simulink model "BMSSOCEstimation"  (R2025b)
settings: Solver=FixedStepDiscrete  StartTime=0.0  StopTime=10000  FixedStep=0.1  RelTol=1e-3
model workspace (MAT data in the model file):
  Battery.SOC_LUT = [0.01 0.02 0.03 0.04 0.05 0.06 0.07 0.08 0.09 0.1 0.11 0.12 0.13 0.14 0.15 0.16 0.17 0.18 0.19 0.2 0.21 0.22 0.23 0.24 0.25 0.26 0.27 0.28 0.29 0.3 0.31 0.32 0.33 0.34 0.35 0.36 0.37 0.38 0.39 0.4 0.41 0.42 0.43 0.44 0.45 0.46 0.47 0.48 0.49 0.5 0.51 0.52 0.53 0.54 0.55 0.56 0.57 0.58 0.59 0.6 0.61 0.62 0.63 0.64 0.65 0.66 0.67 0.68 0.69 0.7 0.71 0.72 0.73 0.74 0.75 0.76 0.77 0.78 0.79 0.8 0.81 0.82 0.83 0.84 0.85 0.86 0.87 0.88 0.89 0.9 0.91 0.92 0.93 0.94 0.95 0.96 0.97 0.98 0.99 1]
  Battery.Temperature_LUT = [-10 0 25 40]
  Battery.Capacity_LUT = [4.04528301887 4.19622641509 4.8 4.73962264151]
  Battery.Em_LUT = [2.67308083891 2.74411674384 2.80408613071 2.86247711994 2.90851059763 2.94904306488 2.9829846776 3.01467102589 3.04031502638 3.06256828113 3.08180972392 3.09994219643 ... (400 elements, 100x4)]
  Battery.R0_LUT = [0.0569026752707 0.0575506938969 0.0576730924021 0.0575627404981 0.0573787336615 0.0571931123197 0.0568199985482 0.056411926464 0.0561974340667 0.0560805640861 0.0557640899305 0.055275807865 ... (400 elements, 100x4)]
  Battery.R1_LUT = [0.0035 0.0035 0.0035 0.0035 0.0035 0.0035 0.0035 0.0035 0.0035 0.0035 0.0035 0.0035 ... (400 elements, 100x4)]
  Battery.C1_LUT = [5000 5000 5000 5000 5000 5000 5000 5000 5000 5000 5000 5000 ... (400 elements, 100x4)]
  Battery.Mass = 0.047
  Battery.ThermalMass = 44
  Battery.R_bleed = 20
  Battery.h_conv = 5
  Battery.cell_area = 0.0037
  Battery.TempInit = 25
  Battery.SOCInit = 0.75
  Battery.Model = 'panasonic ncr18650bd'
  Battery.DischargeCycle_LUT = [1 5 9 13 17 21 25 29 33 37 41 45 49 53 57 61 65 69 73 77 81 85 89 93 97 101 105 109 113 117 121 125 129 133 137 141 145 149 153 157 161 165 169 173 177 181 185 189 193 197 201 205 209 213 217 221 225 229 233 237 241 245 249 253 257 261 265 269 273 277 281 285 289 293 297 301 305 309 313 317]
  Battery.deltaEm_LUT = [0 -0.363115641304 -0.600096647258 -0.689070000839 -0.76773380251 -0.846397604181 -0.926368385458 -0.992711297521 -1.05704974111 -1.12227693902 -1.19018070587 -1.25808447272 -1.31699459748 -1.35876443799 -1.40168267642 -1.44460091485 -1.48751915327 -1.5304373917 -1.57335563013 -1.62198241593 -1.67232184498 -1.71858340023 -1.76179802551 -1.8050126508 -1.84822727608 -1.8917937136 -1.93575272784 -1.97971174208 -2.02367075632 -2.06762977056 -2.11171979109 -2.15588700406 -2.19980020032 -2.24365853098 -2.28751686164 -2.33137519231 -2.37523352297 -2.41909185363 -2.45982559031 -2.49599372373 -2.53216185715 -2.56832999058 -2.604498124 -2.64066625743 -2.67683439085 -2.71300252428 -2.7491706577 -2.78367585394 -2.81632179346 -2.8483348579 -2.88034792233 -2.91236098677 -2.94437405121 -2.97638711564 -3.00840018008 -3.04041324451 -3.07260346059 -3.10359008254 -3.13082308991 -3.15805609728 -3.18528910464 -3.21252211201 -3.23975511938 -3.26698812675 -3.29422113412 -3.32122400938 -3.3463475604 -3.37152613073 -3.39670470105 -3.42188327138 -3.4470618417 -3.47224041203 -3.49938358795 -3.52900276724 -3.55862194653 -3.58824112582 -3.6178603051 -3.64748858268 -3.67711690909 -3.70674523549]
  Battery.deltaCapacity_LUT = [0 -0.860019120059 -1.71332421702 -2.0819400264 -2.45055583577 -2.81917164515 -3.18778745452 -3.48884924257 -3.7808148236 -4.07278040463 -4.36474598566 -4.6567115667 -4.91000721732 -5.08494410056 -5.2598809838 -5.43481786703 -5.60975475027 -5.78469163351 -5.95962851674 -6.13456539998 -6.30950228322 -6.47026795816 -6.62044510558 -6.77062225299 -6.92079940041 -7.07097654783 -7.22115369524 -7.37133084266 -7.52150799007 -7.67168513749 -7.82230984162 -7.97319825819 -8.12408667477 -8.27497509134 -8.42586350792 -8.57675192449 -8.72764034107 -8.87852875764 -9.01789522921 -9.13717923376 -9.25646323831 -9.37574724285 -9.4950312474 -9.61431525195 -9.73359925649 -9.85288326104 -9.97216726558 -10.0914512701 -10.2059878191 -10.3183039593 -10.4306200996 -10.5429362398 -10.65525238 -10.7675685203 -10.8798846605 -10.9922008008 -11.104516941 -11.2125891929 -11.3075699376 -11.4025506823 -11.4975314271 -11.5925121718 -11.6874929166 -11.7824736613 -11.877454406 -11.9716325175 -12.0588579537 -12.1460833899 -12.2333088261 -12.3205342623 -12.4077596986 -12.4949851348 -12.5890165008 -12.6916254178 -12.7942343349 -12.8968432519 -12.999452169 -13.102061086 -13.2046700031 -13.3072789201]
  Battery.cond_thickness = 0.001
  Battery.thermal_conductivity = 205
  Ts = Simulink.Parameter
  Ts.Value = 0.1
  Ts.Complexity = 'real'
  Ts.Dimensions = [1 1]
  Ts.DataType = 'double'
undefined symbols (not defined in the file): DiscIntNeverNeededParam, PlntBattNumCellPar, PlntBattSocInit
libraries: sharedTrackingLibrary x2, simulink x1
settings Model: DataDictionary=VirtualMotoTemplate.sldd  ModifiedByFormat=The MathWorks, Inc.  ExtModeTrigDuration=5  Creator=The MathWorks, Inc.  LastModifiedBy=The MathWorks, Inc.
settings SolverCC: AlgebraicLoopSolver=TrustRegion  PositivePriorityOrder=on  AutoInsertRateTranBlk=on  MaxZcPerStep=1.0
settings DataIOCC: ExternalInput=Battery  SaveOutput=off  SaveTime=off  SignalLoggingName=logsOut
settings OptimizationCC: BlockReduction=off  DefaultParameterBehavior=Inlined  UseFloatMulNetSlope=on  DefaultUnderspecifiedDataType=single  OptimizeBlockIOStorage=off  ReuseModelBlockBuffer=off  EnhancedBackFolding=on  PassReuseOutputArgsThreshold=0.0  ZeroExternalMemoryAtStartup=off  ZeroInternalMemoryAtStartup=off  EfficientFloat2IntCast=on  MaxStackSize=64  OptimizeBlockOrder=speed  DifferentSizesBufferReuse=on
settings DebuggingCC: SignalInfNanChecking=error  SaveWithParameterizedLinksMsg=none  CheckExecutionContextPreStartOutputMsg=on  IntegerOverflowMsg=error  ParameterPrecisionLossMsg=none  ParameterTunabilityLossMsg=error  UnconnectedInputMsg=warning  UnconnectedOutputMsg=warning  UnconnectedLineMsg=warning  AssertControl=DisableAll  PregeneratedLibrarySubsystemCodeDiagnostic=none  SFUnexpectedBacktrackingDiag=warning  SFNoUnconditionalDefaultTransitionDiag=warning  SFExecutionAtInitializationDiag=none  ArithmeticOperatorsInVariantConditions=warning
settings HardwareCC: ProdBitPerLong=64.0  ProdLongLongMode=on  ProdHWDeviceType=Intel->x86-64 (Linux 64)
settings ModelReferenceCC: EnableRefExpFcnMdlSchedulingChecks=on  ModelReferenceNumInstancesAllowed=Single  PropagateSignalLabelsOutOfModel=off
settings SFSimCC: SimUseLocalCustomCode=off  MATLABDynamicMemAlloc=off  CustomCodeUndefinedFunction=UseInterfaceOnly
settings RTWCC: GenerateReport=on  RTWUseLocalCustomCode=off  Toolchain=Simulink Real-Time Toolchain  BuildConfiguration=Faster Runs  TargetLang=C++  GPUComputeCapability=3.5  DLArmComputeVersion=19.05
settings CodeAppCC: ForceParamTrailComments=on  MaxIdLength=51.0  OperatorAnnotations=on  MangleLength=4.0
settings GRTTargetCC: TargetLangStandard=C++03 (ISO)  CodeInterfacePackaging=C++ class  SubcomponentCodeInterfacePackaging=C++ class
settings ConfigComp: CovMetricSettings=dcw  CovSaveCumulativeToWorkspaceVar=on  CovSaveSingleToWorkspaceVar=on  CovExternalEMLEnable=off  CovSFcnEnable=off  DVMode=DesignErrorDetection  DVMaxProcessTime=7000.0  DVMaxTestCaseSteps=10000.0  DVTestSuiteOptimization=Auto  DVAbsoluteTolerance=1.0e-5  DVDefectChecker=on  DVDetectDeadLogic=on  DVDetectIntegerOverflow=off  DVMaxViolationSteps=20.0  DVHarnessSource=Signal Editor  DVRebuildModelRepresentation=Always  DVActiveTab=0.0

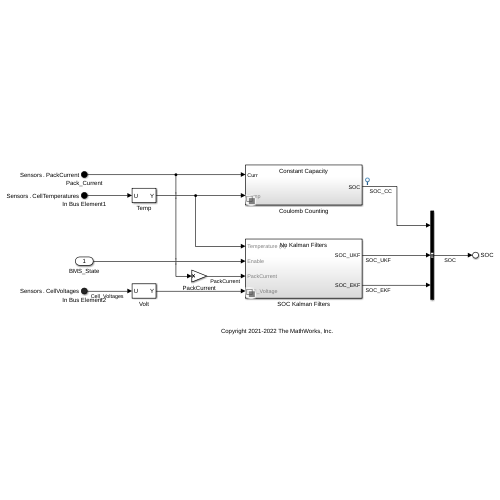
[thumbnail: Simulink's stored preview of the top-level diagram]
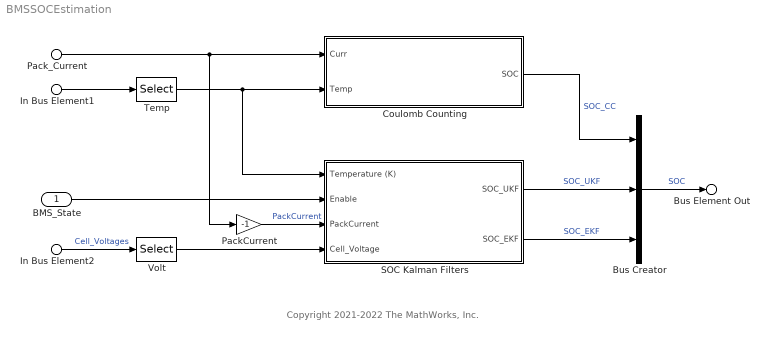
== system BMSSOCEstimation ==
  note: Copyright 2021-2022 The MathWorks, Inc.
  BMS_State : Inport
  In Bus Element2 : Inport  Port=2  PortName=Sensors  Element=CellVoltages
  Pack_Current : Inport  Port=2  PortName=Sensors  Element=PackCurrent
  In Bus Element1 : Inport  Port=2  PortName=Sensors  Element=CellTemperatures
  Bus Creator : BusCreator  Inputs=3
  Coulomb Counting : Subsystem  Variant=on  VariantControlMode=label  VariantControl=SocAlgo==1  LabelModeActiveChoice=Constant Capacity
  PackCurrent : Gain  Gain=-1
  SOC Kalman Filters : Subsystem  Variant=on  VariantControlMode=label  VariantControl=Choice  LabelModeActiveChoice=No Kalman Filters
  Temp : Selector  InputPortWidth=PlntBattNumCellSer  IndexOptions=Index vector (dialog)  Indices=1  OutputSizes=1
  Volt : Selector  InputPortWidth=PlntBattNumCellSer  IndexOptions=Index vector (dialog)  Indices=1  OutputSizes=1
  Bus Element Out : Outport  PortName=SOC
  wires:
  Bus Creator/1 -> Bus Element Out/1  "SOC"
  In Bus Element2/1 -> Volt/1  "Cell_Voltages"
  Temp/1 -> Coulomb Counting/2(Temp), SOC Kalman Filters/1(Temperature (K))
  Pack_Current/1 -> Coulomb Counting/1(Curr), PackCurrent/1
  In Bus Element1/1 -> Temp/1
  Coulomb Counting/1(SOC) -> Bus Creator/1  "SOC_CC"
  BMS_State/1 -> SOC Kalman Filters/2(Enable)
  PackCurrent/1 -> SOC Kalman Filters/3(PackCurrent)  "PackCurrent"
  Volt/1 -> SOC Kalman Filters/4(Cell_Voltage)
  SOC Kalman Filters/1(SOC_UKF) -> Bus Creator/2  "SOC_UKF"
  SOC Kalman Filters/2(SOC_EKF) -> Bus Creator/3  "SOC_EKF"

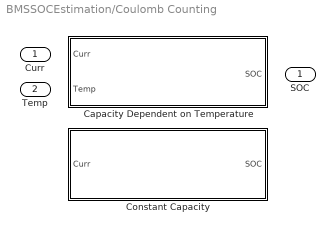
== system BMSSOCEstimation/Coulomb Counting ==
  Curr : Inport
  Temp : Inport  Port=2
  Capacity Dependent on Temperature : Subsystem  VariantControl=Capacity Dependent on Temperature
  Constant Capacity : Subsystem  VariantControl=Constant Capacity
  SOC : Outport

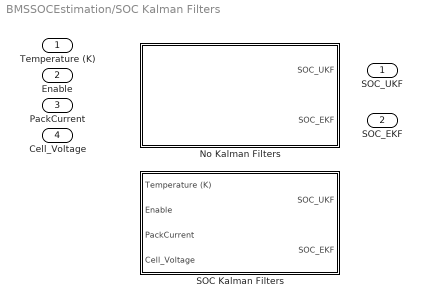
== system BMSSOCEstimation/SOC Kalman Filters ==
  Temperature (K) : Inport
  Enable : Inport  Port=2
  PackCurrent : Inport  Port=3
  Cell_Voltage : Inport  Port=4
  No Kalman Filters : Subsystem  VariantControl=No Kalman Filters
  SOC Kalman Filters : Subsystem  InitFcn=|  VariantControl=SOC Kalman Filters
      | if ~license('test', 'identification_toolbox') 
      |   error(['Block' gcb ' Requires System Identification Toolbox']) 
      | end 
      | 
      | if ~license('test', 'control_toolbox') 
      |     error(['Block' gcb ' Requires Control System Toolbox']) 
      | end
  SOC_UKF : Outport
  SOC_EKF : Outport  Port=2

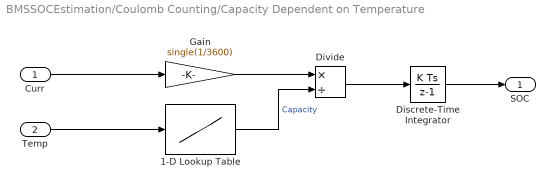
== system BMSSOCEstimation/Coulomb Counting/Capacity Dependent on Temperature ==
  Curr : Inport
  Temp : Inport  Port=2
  1-D Lookup Table : Lookup_n-D  NumberOfTableDimensions=1  BreakpointsForDimension1=single(Battery(1).Temperature_LUT)  Table=single(Battery(1).Capacity_LUT)*PlntBattNumCellPar  InternalRulePriority=Speed  RndMeth=Simplest
  Discrete-Time Integrator : DiscreteIntegrator  InitialCondition=single(PlntBattSocInit)  SampleTime=-1  LimitOutput=on  UpperSaturationLimit=1  LowerSaturationLimit=0  ICPrevOutput=DiscIntNeverNeededParam  ICPrevScaledInput=DiscIntNeverNeededParam
  Divide : Product  Inputs=*/
  Gain : Gain  Gain=single(1/3600)
  SOC : Outport  VectorParamsAs1DForOutWhenUnconnected=off
  wires:
  Discrete-Time Integrator/1 -> SOC/1
  Curr/1 -> Gain/1
  Gain/1 -> Divide/1
  Divide/1 -> Discrete-Time Integrator/1
  1-D Lookup Table/1 -> Divide/2  "Capacity"
  Temp/1 -> 1-D Lookup Table/1

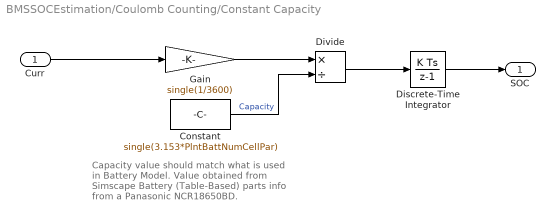
== system BMSSOCEstimation/Coulomb Counting/Constant Capacity ==
  note: Capacity value should match
      | what is used in Battery Model.
      | Value obtained from Simscape
      | Battery (Table-Based) parts info
      | from a Panasonic NCR18650BD.
  Curr : Inport
  Constant : Constant  Value=single(3.153*PlntBattNumCellPar)  SampleTime=-1
  Discrete-Time Integrator : DiscreteIntegrator  InitialCondition=single(PlntBattSocInit)  SampleTime=-1  LimitOutput=on  UpperSaturationLimit=1  LowerSaturationLimit=0  ICPrevOutput=DiscIntNeverNeededParam  ICPrevScaledInput=DiscIntNeverNeededParam
  Divide : Product  Inputs=*/
  Gain : Gain  Gain=single(1/3600)
  SOC : Outport  VectorParamsAs1DForOutWhenUnconnected=off
  wires:
  Constant/1 -> Divide/2  "Capacity"
  Divide/1 -> Discrete-Time Integrator/1
  Gain/1 -> Divide/1
  Curr/1 -> Gain/1
  Discrete-Time Integrator/1 -> SOC/1

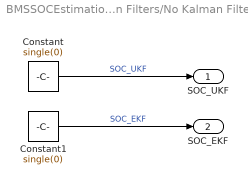
== system BMSSOCEstimation/SOC Kalman Filters/No Kalman Filters ==
  Constant : Constant  Value=single(0)  SampleTime=-1
  Constant1 : Constant  Value=single(0)  SampleTime=-1
  SOC_UKF : Outport
  SOC_EKF : Outport  Port=2
  wires:
  Constant/1 -> SOC_UKF/1  "SOC_UKF"
  Constant1/1 -> SOC_EKF/1  "SOC_EKF"

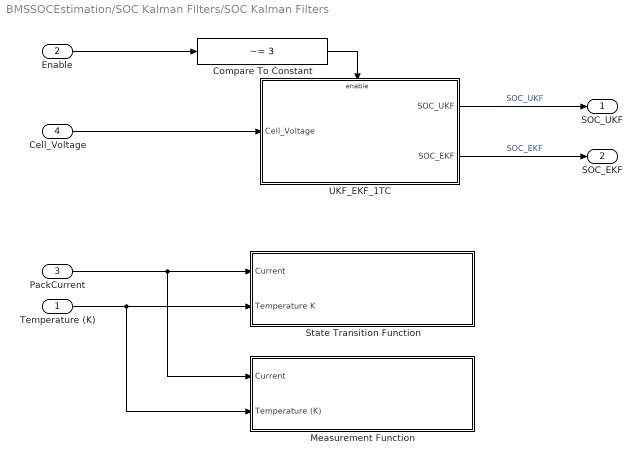
== system BMSSOCEstimation/SOC Kalman Filters/SOC Kalman Filters ==
  Temperature (K) : Inport
  Enable : Inport  Port=2
  PackCurrent : Inport  Port=3
  Cell_Voltage : Inport  Port=4
  Compare To Constant : simulink/Logic and Bit Operations/Compare To Constant  relop=~=  const=3  OutDataTypeStr=boolean
  Measurement Function : Subsystem  TreatAsAtomicUnit=on
  State Transition Function : Subsystem  TreatAsAtomicUnit=on
  UKF_EKF_1TC : Subsystem  VariantControl=CellType==1
  SOC_UKF : Outport
  SOC_EKF : Outport  Port=2
  wires:
  Cell_Voltage/1 -> UKF_EKF_1TC/1(Cell_Voltage)
  UKF_EKF_1TC/2(SOC_EKF) -> SOC_EKF/1  "SOC_EKF"
  Temperature (K)/1 -> State Transition Function/2(Temperature K), Measurement Function/2(Temperature (K))
  Compare To Constant/1 -> UKF_EKF_1TC/Enable
  UKF_EKF_1TC/1(SOC_UKF) -> SOC_UKF/1  "SOC_UKF"
  PackCurrent/1 -> State Transition Function/1(Current), Measurement Function/1(Current)
  Enable/1 -> Compare To Constant/1

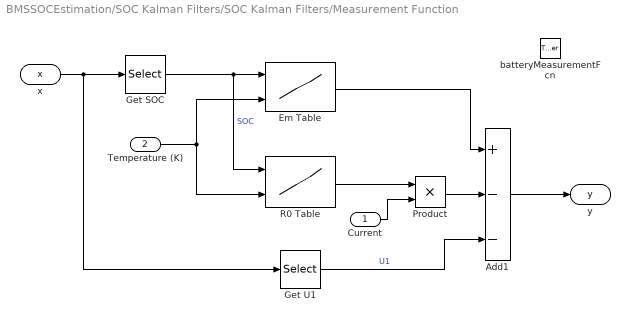
== system BMSSOCEstimation/SOC Kalman Filters/SOC Kalman Filters/Measurement Function ==
  Current : Inport
  Temperature (K) : Inport  Port=2
  batteryMeasurementFcn : TriggerPort  TriggerType=function-call  IsSimulinkFunction=on  FunctionName=batteryMeasurementFcn  VariantControl=Variant
  Add1 : Sum  Inputs=+--
  Em Table : Lookup_n-D  BreakpointsForDimension1=Battery.SOC_LUT  BreakpointsForDimension2=Battery.Temperature_LUT  BeginIndexSearchUsingPreviousIndexResult=on  Table=Battery.Em_LUT  ExtrapMethod=Clip  InternalRulePriority=Speed  RndMeth=Simplest
      settings: InputPortMap=u0,u1
  Get SOC : Selector  InputPortWidth=2  IndexOptions=Index vector (dialog)  Indices=[1]  OutputSizes=1
  Get U1 : Selector  InputPortWidth=2  IndexOptions=Index vector (dialog)  Indices=2  OutputSizes=1
  Product : Product
  R0 Table : Lookup_n-D  BreakpointsForDimension1=Battery.SOC_LUT  BreakpointsForDimension2=Battery.Temperature_LUT  BeginIndexSearchUsingPreviousIndexResult=on  Table=Battery.R0_LUT  ExtrapMethod=Clip  InternalRulePriority=Speed  RndMeth=Simplest
      settings: InputPortMap=u0,u1
  x : ArgIn  DisableCoverage=on  OutDataTypeStr=single  PortDimensions=2  ArgumentName=x
  y : ArgOut  DisableCoverage=on  OutDataTypeStr=single  ArgumentName=y
  wires:
  Get U1/1 -> Add1/3  "U1"
  Product/1 -> Add1/2
  Current/1 -> Product/2
  R0 Table/1 -> Product/1
  Temperature (K)/1 -> Em Table/2, R0 Table/2
  Add1/1 -> y/1
  Em Table/1 -> Add1/1
  Get SOC/1 -> Em Table/1, R0 Table/1  "SOC"
  x/1 -> Get SOC/1, Get U1/1

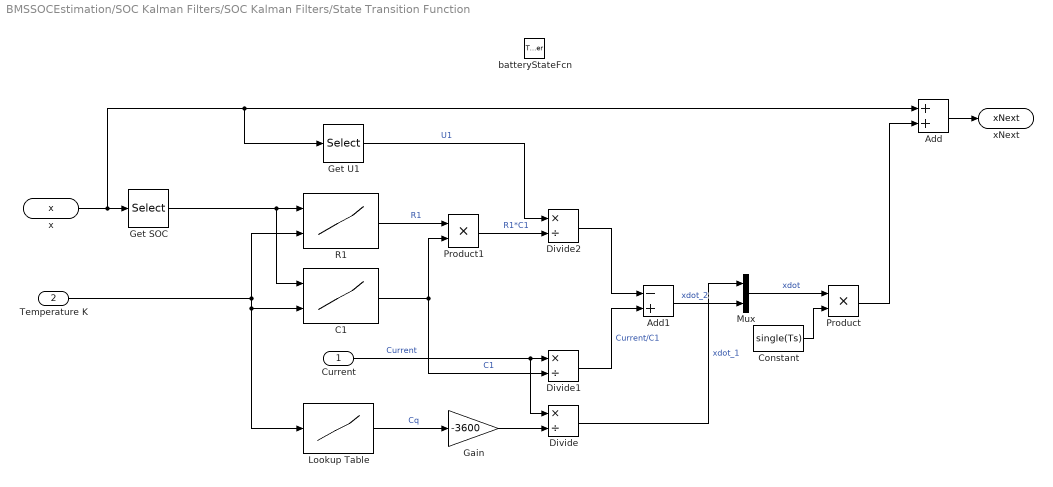
== system BMSSOCEstimation/SOC Kalman Filters/SOC Kalman Filters/State Transition Function ==
  Current : Inport
  Temperature K : Inport  Port=2
  batteryStateFcn : TriggerPort  TriggerType=function-call  IsSimulinkFunction=on  FunctionName=batteryStateFcn  VariantControl=Variant
  Add : Sum
  Add1 : Sum  Inputs=-+
  C1 : Lookup_n-D  BreakpointsForDimension1=Battery.SOC_LUT  BreakpointsForDimension2=Battery.Temperature_LUT  BeginIndexSearchUsingPreviousIndexResult=on  Table=Battery.C1_LUT  ExtrapMethod=Clip  InternalRulePriority=Speed  RndMeth=Simplest
      settings: InputPortMap=u0,u1
  Constant : Constant  Value=single(Ts)  OutDataTypeStr=single
  Divide : Product  Inputs=*/
  Divide1 : Product  Inputs=*/
  Divide2 : Product  Inputs=*/
  Gain : Gain  Gain=-3600
  Get SOC : Selector  InputPortWidth=2  IndexOptions=Index vector (dialog)  Indices=1  OutputSizes=1
  Get U1 : Selector  InputPortWidth=2  IndexOptions=Index vector (dialog)  Indices=2  OutputSizes=1
  Lookup Table : Lookup_n-D  NumberOfTableDimensions=1  BreakpointsForDimension1=Battery.Temperature_LUT  BeginIndexSearchUsingPreviousIndexResult=on  Table=Battery.Capacity_LUT  InternalRulePriority=Speed  RndMeth=Simplest
  Mux : Mux  Inputs=2
  Product : Product  OutDataTypeStr=single
  Product1 : Product
  R1 : Lookup_n-D  BreakpointsForDimension1=Battery.SOC_LUT  BreakpointsForDimension2=Battery.Temperature_LUT  BeginIndexSearchUsingPreviousIndexResult=on  Table=Battery.R1_LUT  ExtrapMethod=Clip  InternalRulePriority=Speed  RndMeth=Simplest
      settings: InputPortMap=u0,u1
  x : ArgIn  DisableCoverage=on  OutDataTypeStr=single  PortDimensions=2  ArgumentName=x
  xNext : ArgOut  DisableCoverage=on  OutDataTypeStr=single  PortDimensions=2  ArgumentName=xNext
  wires:
  Lookup Table/1 -> Gain/1  "Cq"
  Product/1 -> Add/2
  Constant/1 -> Product/2
  Current/1 -> Divide1/1, Divide/1  "Current"
  Get SOC/1 -> C1/1, R1/1
  Temperature K/1 -> Lookup Table/1, C1/2, R1/2
  Add/1 -> xNext/1
  x/1 -> Add/1, Get U1/1, Get SOC/1
  Gain/1 -> Divide/2
  Divide/1 -> Mux/1  "xdot_1"
  Get U1/1 -> Divide2/1  "U1"
  Product1/1 -> Divide2/2  "R1*C1"
  R1/1 -> Product1/1  "R1"
  C1/1 -> Product1/2, Divide1/2  "C1"
  Divide1/1 -> Add1/2  "Current/C1"
  Divide2/1 -> Add1/1
  Add1/1 -> Mux/2  "xdot_2"
  Mux/1 -> Product/1  "xdot"

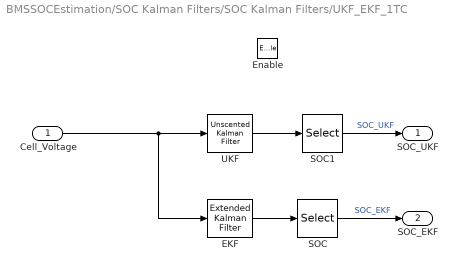
== system BMSSOCEstimation/SOC Kalman Filters/SOC Kalman Filters/UKF_EKF_1TC ==
  Cell_Voltage : Inport
  Enable : EnablePort
  EKF : sharedTrackingLibrary/Extended Kalman Filter  StateTransitionFcn=batteryStateFcn  HasStateTransitionJacobianFcn=off  HasAdditiveProcessNoise=Additive  ProcessNoise=1e-10*eye(2)  HasTimeVaryingProcessNoise=off  HasStateTransitionFcnExtraArgument=0  InitialState=[single(PlntBattSocInit+0.05); 0;]  InitialStateCovariance=[1e-5 1]  MeasurementFcn1=batteryMeasurementFcn  HasMeasurementJacobianFcn1=off  HasMeasurementEnablePort1=off  HasAdditiveMeasurementNoise1=Additive  MeasurementNoise1=1e-1  HasTimeVaryingMeasurementNoise1=off  HasMeasurementFcnExtraArgument1=0  HasMeasurementWrapping1=off  MeasurementFcn2=myMeasurementFcn  HasMeasurementJacobianFcn2=off  HasMeasurementEnablePort2=off  HasAdditiveMeasurementNoise2=Additive  MeasurementNoise2=1  HasTimeVaryingMeasurementNoise2=off  HasMeasurementFcnExtraArgument2=0  HasMeasurementWrapping2=off  MeasurementFcn3=myMeasurementFcn  HasMeasurementJacobianFcn3=off  HasMeasurementEnablePort3=off  HasAdditiveMeasurementNoise3=Additive  MeasurementNoise3=1  HasTimeVaryingMeasurementNoise3=off  HasMeasurementFcnExtraArgument3=0  HasMeasurementWrapping3=off  MeasurementFcn4=myMeasurementFcn  HasMeasurementJacobianFcn4=off  HasMeasurementEnablePort4=off  HasAdditiveMeasurementNoise4=Additive  MeasurementNoise4=1  HasTimeVaryingMeasurementNoise4=off  HasMeasurementFcnExtraArgument4=0  HasMeasurementWrapping4=off  MeasurementFcn5=myMeasurementFcn  HasMeasurementJacobianFcn5=off  HasMeasurementEnablePort5=off  HasAdditiveMeasurementNoise5=Additive  MeasurementNoise5=1  HasTimeVaryingMeasurementNoise5=off  HasMeasurementFcnExtraArgument5=0  HasMeasurementWrapping5=off  EnableMultirate=off  StateTransitionFcnSampleTime=1  MeasurementFcn1SampleTime=1  MeasurementFcn2SampleTime=1  MeasurementFcn3SampleTime=1  MeasurementFcn4SampleTime=1  MeasurementFcn5SampleTime=1  UseCurrentEstimator=on  OutputStateCovariance=off  DataType=single  SampleTime=Ts  NumberOfMeasurements=1
  SOC : Selector  InputPortWidth=2  IndexOptions=Index vector (dialog)  Indices=1  OutputSizes=1
  SOC1 : Selector  InputPortWidth=2  IndexOptions=Index vector (dialog)  Indices=1  OutputSizes=1
  UKF : sharedTrackingLibrary/Unscented Kalman Filter  StateTransitionFcn=batteryStateFcn  HasAdditiveProcessNoise=Additive  ProcessNoise=1e-10*eye(2)  HasTimeVaryingProcessNoise=off  HasStateTransitionFcnExtraArgument=0  InitialState=[single(PlntBattSocInit+0.05); 0;]  InitialStateCovariance=[1e-5 1]  Alpha=1  Beta=2  Kappa=1  MeasurementFcn1=batteryMeasurementFcn  HasMeasurementEnablePort1=off  HasAdditiveMeasurementNoise1=Additive  MeasurementNoise1=0.1  HasTimeVaryingMeasurementNoise1=off  HasMeasurementFcnExtraArgument1=0  HasMeasurementWrapping1=off  MeasurementFcn2=myMeasurementFcn  HasMeasurementEnablePort2=off  HasAdditiveMeasurementNoise2=Additive  MeasurementNoise2=1  HasTimeVaryingMeasurementNoise2=off  HasMeasurementFcnExtraArgument2=0  HasMeasurementWrapping2=off  MeasurementFcn3=myMeasurementFcn  HasMeasurementEnablePort3=off  HasAdditiveMeasurementNoise3=Additive  MeasurementNoise3=1  HasTimeVaryingMeasurementNoise3=off  HasMeasurementFcnExtraArgument3=0  HasMeasurementWrapping3=off  MeasurementFcn4=myMeasurementFcn  HasMeasurementEnablePort4=off  HasAdditiveMeasurementNoise4=Additive  MeasurementNoise4=1  HasTimeVaryingMeasurementNoise4=off  HasMeasurementFcnExtraArgument4=0  HasMeasurementWrapping4=off  MeasurementFcn5=myMeasurementFcn  HasMeasurementEnablePort5=off  HasAdditiveMeasurementNoise5=Additive  MeasurementNoise5=1  HasTimeVaryingMeasurementNoise5=off  HasMeasurementFcnExtraArgument5=0  HasMeasurementWrapping5=off  EnableMultirate=off  StateTransitionFcnSampleTime=-1  MeasurementFcn1SampleTime=-1  MeasurementFcn2SampleTime=-1  MeasurementFcn3SampleTime=-1  MeasurementFcn4SampleTime=-1  MeasurementFcn5SampleTime=-1  UseCurrentEstimator=on  OutputStateCovariance=off  DataType=single  SampleTime=Ts  NumberOfMeasurements=1
  SOC_UKF : Outport  VectorParamsAs1DForOutWhenUnconnected=off
  SOC_EKF : Outport  Port=2  VectorParamsAs1DForOutWhenUnconnected=off
  wires:
  UKF/1 -> SOC1/1
  Cell_Voltage/1 -> UKF/1, EKF/1
  SOC1/1 -> SOC_UKF/1  "SOC_UKF"
  EKF/1 -> SOC/1
  SOC/1 -> SOC_EKF/1  "SOC_EKF"
